simulink model "d_Animation"  (R2020b)
settings: Solver=VariableStepAuto  StartTime=0.0  StopTime=inf  RelTol=1e-3
libraries: vrlib x6
settings Model: EnablePacing=on  Creator=eric  LastModifiedBy=KNguyen

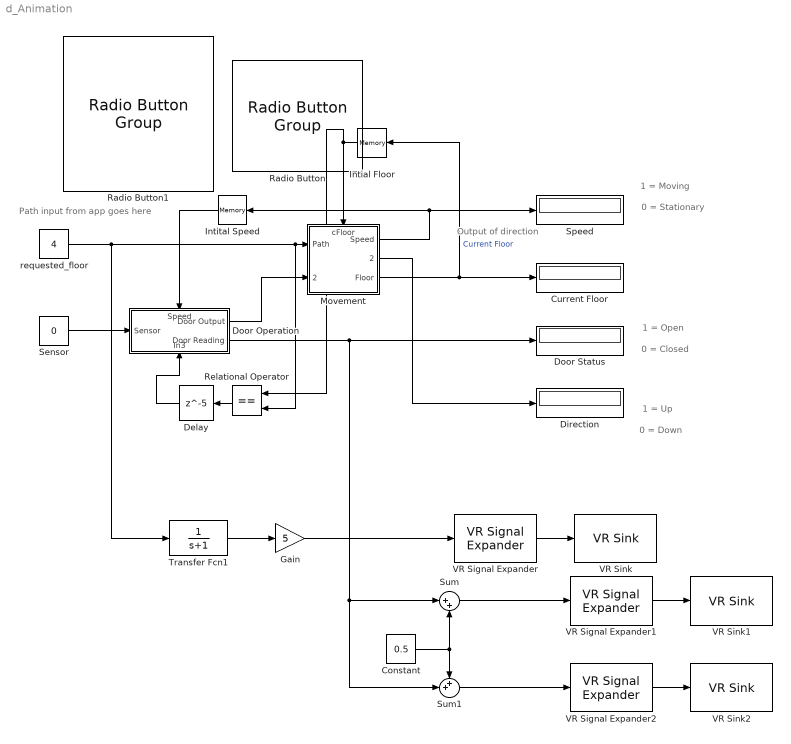
== system d_Animation ==
  note: 0 = Closed
  note: 1 = Open
  note: 0 = Stationary
  note: 1 = Moving
  note: 0 = Down
  note: 1 = Up
  note: Output of direction
  note: Path input from app goes here
  Constant : Constant  Value=0.5
  Current Floor : Display
  Delay : Delay  DelayLength=5  DelayLengthUpperLimit=1  InitialCondition=5
  Direction : Display
  Door Operation : Subsystem
      settings: PortSchema="{\"entries\":[{\"content\":{\"sides\":[{\"content\":{\"connectorIds\":[\"In1\"]},\"type\":\"ConnectorPlacement.EquallySpacedRectSide\",\"uuid\":\"30977b0a-2af7-4c61-bebb-4ec80410b903\"},{\"content\":{\"connectorIds\":[\"Out1\",\"Out2\"],\"side\":\"RIGHT\"},\"type\":\"ConnectorPlacement.EquallySpacedRectSide\",\"uuid\":\"323388e5-4c35-430e-8d9e-2a05895b747e\"},{\"content\":{\"connectorIds\":[\"In2\"],\"side\":\"TOP\"},\"type\":\"ConnectorPlacement.EquallySpacedRectSide\",\"uuid\":\"9d5d1b04-f04c-4d1c-b5e3-f520ce15ffef\"},{\"content\":{\"connectorIds\":[\"In3\"],\"side\":\"BOTTOM\"},\"type\":\"ConnectorPlacement.EquallySpacedRectSide\",\"uuid\":\"a2796d79-cbcd-43fd-84cb-bc57d429544b\"},{\"content\":{\"connectorIds\":[],\"side\":\"HIDDEN\"},\"type\":\"ConnectorPlacement.EquallySpacedRectSide\",\"uuid\":\"d7ca2218-6b24-4bda-a0e6-55c9b81b1772\"}]},\"type\":\"ConnectorPlacement.EquallySpacedConnector\",\"uuid\":\"8cf9c2d5-6e60-4b33-b84b-36b0ae7fd4c7\"}],\"packageUris\":[\"http://schema.mathworks.com/mf0/Connector/R2020b\"],\"version\":\"1.0\"}"
  Door Status : Display
      settings: Format=decimal (Stored Integer)
  Gain : Gain  Gain=5
  Intial Floor : Memory
  Intital Speed : Memory
  Movement : Stateflow chart  TreatAsAtomicUnit=on
      settings: PortSchema="{\"entries\":[{\"content\":{\"sides\":[{\"content\":{\"connectorIds\":[\"In3\",\"In2\"]},\"type\":\"ConnectorPlacement.EquallySpacedRectSide\",\"uuid\":\"723fcccf-a5ea-4524-a847-31e47b2c7577\"},{\"content\":{\"connectorIds\":[\"Out1\",\"Out2\",\"Out3\"],\"side\":\"RIGHT\"},\"type\":\"ConnectorPlacement.EquallySpacedRectSide\",\"uuid\":\"c79bb0ca-7135-417f-bf20-d4a9209b0782\"},{\"content\":{\"connectorIds\":[\"In1\"],\"side\":\"TOP\"},\"type\":\"ConnectorPlacement.EquallySpacedRectSide\",\"uuid\":\"4a8db4cf-0e92-4abd-a983-fa8b3d66675d\"},{\"content\":{\"connectorIds\":[],\"side\":\"HIDDEN\"},\"type\":\"ConnectorPlacement.EquallySpacedRectSide\",\"uuid\":\"59d7251f-75ad-48da-8ece-7fda6e08ec45\"}]},\"type\":\"ConnectorPlacement.EquallySpacedConnector\",\"uuid\":\"c629af32-1ebf-4e2d-97c9-9fb50af07127\"}],\"packageUris\":[\"http://schema.mathworks.com/mf0/Connector/R2020b\"],\"version\":\"1.0\"}"
  Radio Button : RadioButtonGroup  SelectedLabel=No Obstruction  ButtonGroupName=Sensor
      settings: Values={{'No Obstruction', 'Obstruction'}, [0 1]}
  Radio Button1 : RadioButtonGroup  SelectedLabel=4  ButtonGroupName=Floor
      settings: Values={{'0', '1', '2', '3', '4', '5'}, [0 1 2 3 4 5]}
  Relational Operator : RelationalOperator  Operator===  OutDataTypeStr=boolean  RndMeth=Simplest
  Sensor : Constant  Value=0
  Speed : Display
      settings: Format=decimal (Stored Integer)
  Sum : Sum  Inputs=|++
  Sum1 : Sum  Inputs=++|
  Transfer Fcn1 : TransferFcn  Denominator=[1 1]
  VR Signal Expander : vrlib/VR Signal Expander  outwidth=3  outidx=[2]
  VR Signal Expander1 : vrlib/VR Signal Expander  outwidth=3  outidx=[1]
  VR Signal Expander2 : vrlib/VR Signal Expander  outwidth=3  outidx=[1]
  VR Sink : vrlib/VR Sink  InstantiateOnLoad=on  SampleTime=0.01  ViewEnable=on  RemoteChange=off  RemoteView=off  FieldsWritten=box.translation.3.1.1.double  WorldFileName=elevator model.x3d  AutoView=off  VideoDimensions=[]  AllowVariableSize=off
  VR Sink1 : vrlib/VR Sink  InstantiateOnLoad=on  SampleTime=0.01  ViewEnable=on  RemoteChange=off  RemoteView=off  FieldsWritten=Door_L.translation.3.1.1.double  WorldFileName=elevator model.x3d  AutoView=off  VideoDimensions=[]  AllowVariableSize=off
  VR Sink2 : vrlib/VR Sink  InstantiateOnLoad=on  SampleTime=0.01  ViewEnable=on  RemoteChange=off  RemoteView=off  FieldsWritten=Door_R.translation.3.1.1.double  WorldFileName=elevator model.x3d  AutoView=off  VideoDimensions=[]  AllowVariableSize=off
  requested_floor : Constant  Value=4
  wires:
  Movement/3(Floor) -> Current Floor/1, Intial Floor/1  "Current Floor"
  Movement/1(Speed) -> Intital Speed/1, Speed/1
  Door Operation/1(Door Output) -> Movement/2(Door_Output)
  Intial Floor/1 -> Movement/1(cFloor), Relational Operator/1
  Intital Speed/1 -> Door Operation/2(Speed)
  requested_floor/1 -> Transfer Fcn1/1, Relational Operator/2, Movement/3(Path)
  Sensor/1 -> Door Operation/1(Sensor)
  Movement/2(Direction) -> Direction/1
  Delay/1 -> Door Operation/3(In3)
  Constant/1 -> Sum1/1, Sum/2
  VR Signal Expander1/1 -> VR Sink1/1
  VR Signal Expander2/1 -> VR Sink2/1
  Gain/1 -> VR Signal Expander/1
  VR Signal Expander/1 -> VR Sink/1
  Sum/1 -> VR Signal Expander1/1
  Transfer Fcn1/1 -> Gain/1
  Sum1/1 -> VR Signal Expander2/1
  Door Operation/2(Door Reading) -> Door Status/1, Sum1/2, Sum/1
  Relational Operator/1 -> Delay/1

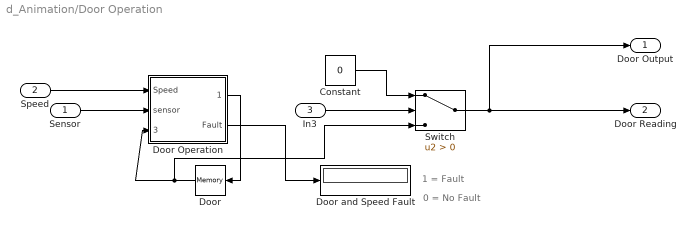
== system d_Animation/Door Operation ==
  note: 0 = No Fault
  note: 1 = Fault
  Sensor : Inport
  Speed : Inport  Port=2  OutMin=0  OutMax=2  OutDataTypeStr=double
  In3 : Inport  Port=3
  Constant : Constant  Value=0
  Door : Memory  InitialCondition=1  InheritSampleTime=on  LinearizeMemory=on
  Door Operation : Stateflow chart  TreatAsAtomicUnit=on
      settings: PortSchema="{\"entries\":[{\"content\":{\"sides\":[{\"content\":{\"connectorIds\":[\"In2\",\"In1\",\"In3\"]},\"type\":\"ConnectorPlacement.EquallySpacedRectSide\",\"uuid\":\"31e92d3c-0266-4042-9cc0-73e2fa5475a5\"},{\"content\":{\"connectorIds\":[\"Out1\",\"Out2\"],\"side\":\"RIGHT\"},\"type\":\"ConnectorPlacement.EquallySpacedRectSide\",\"uuid\":\"0ce7aa6e-b975-49b3-b309-422d5642910d\"},{\"content\":{\"connectorIds\":[],\"side\":\"TOP\"},\"type\":\"ConnectorPlacement.EquallySpacedRectSide\",\"uuid\":\"d77baac7-bcfc-4c97-8f5f-a05c60ec2b96\"},{\"content\":{\"connectorIds\":[],\"side\":\"HIDDEN\"},\"type\":\"ConnectorPlacement.EquallySpacedRectSide\",\"uuid\":\"7d61dd79-ac27-4838-8e0e-1c25083bca29\"}]},\"type\":\"ConnectorPlacement.EquallySpacedConnector\",\"uuid\":\"ed20ea32-9081-4fe8-8264-861068f1e86e\"}],\"packageUris\":[\"http://schema.mathworks.com/mf0/Connector/R2020b\"],\"version\":\"1.0\"}"
  Door and Speed Fault : Display
  Switch : Switch  Criteria=u2 > Threshold
  Door Output : Outport
  Door Reading : Outport  Port=2
  wires:
  Speed/1 -> Door Operation/2(Speed)
  Sensor/1 -> Door Operation/1(sensor)
  Door/1 -> Switch/3, Door Operation/3(Door_initial)
  Door Operation/2(Fault) -> Door and Speed Fault/1
  Switch/1 -> Door Output/1, Door Reading/1
  Door Operation/1(Door_output) -> Door/1
  Constant/1 -> Switch/1
  In3/1 -> Switch/2

== stateflow chart d_Animation/Door Operation/Door Operation ==
  state Idle
    en:
    Speed;
    sensor;
    Door =Door_initial;
    Fault = 0;
  state Arrving
    exit:
    Door= 1;
  state Fault [commented out]
    en:
    Door=0;
    Speed=0;
    Fault=1;
  state Door_Output
    en:
    after(5,sec);
  state Obstacle_detection
    en:
    sensor;
    after(2,sec)
  state Leaving
    exit:
    Door= 0;
  note: door open ==1
  Door_Output -> Idle : [after(1,sec)]
  (default) -> Idle
  Idle -> Arrving [order 1] : [Door==0 & Speed==0] %end of path
  Arrving -> Door_Output : {Door_output=1}
  Idle -> Fault [commented out] : [Door==1& Speed > 0]
  Fault -> Idle [commented out] : [Door==0 & Speed==0]
  Idle -> Obstacle_detection [order 2] : [Door==1 & Speed==0]%start of path
  Leaving -> Door_Output : {Door_output=0}
  Obstacle_detection -> Leaving [order 1] : [sensor==0]
  Obstacle_detection -> Obstacle_detection [order 2] : [sensor==1]
  data: sensor input; Door_output output; Speed input; Door local; Door_initial input; Fault output

== stateflow chart d_Animation/Movement ==
  state Idle
    Floor;
    en:
    Action=Path;
    Floor = cFloor;
    exit:
  state Up
    en:
    Speed = 1;
    Direction = 1;
    Floor = Floor +1;
    during:
    motor=1;
    after(3,sec)
    motor= 0
  state Door_Trigger
    during:
    after(2.5,sec)
  state Down
    en:
    Speed = 1;
    Direction = 0;
    Floor = Floor -1;
    during:
    motor=1;
    after(3,sec)
    motor= 0
  Idle -> Door_Trigger [order 4] : [Action==Floor]{Door_Output==1}
  Door_Trigger -> Idle [order 1] : [Door_Output == 0]
  (default) -> Idle
  Idle -> Idle [order 3] : [Action==Floor]
  Idle -> Up [order 1] : [Action>Floor]
  Door_Trigger -> Door_Trigger [order 2] : [Door_Output==1]
  Up -> Door_Trigger [order 1] : [Action==Floor]{Speed=0}
  Idle -> Down [order 2] : [Action<Floor]
  Down -> Door_Trigger [order 2] : [Action==Floor]{Speed=0}
  Up -> Up [order 2] : [Floor~=Action]
  Down -> Down [order 1] : [Floor~=Action]
  data: cFloor input; Speed output; Door_Output input; Path input; Action local; motor local; Direction output; Floor output
